simulink model "LQR_Controller"  (R2025a)
settings: Solver=VariableStepAuto  StartTime=0.0  StopTime=10.0  RelTol=1e-3
settings Model: Creator=xing2  LastModifiedBy=xing2

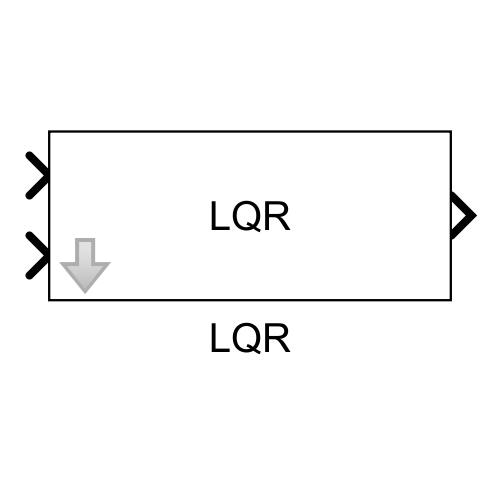
[thumbnail: Simulink's stored preview of the top-level diagram]
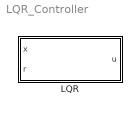
== system LQR_Controller ==
  LQR : Subsystem  mask{K_vec=[3 1], Ki=0, UL=10, LL=-10}
      mask prompts: K_vec "K vector"; Ki "Ki (integral)"; UL "Upper Limit"; LL "Lower Limit"
      mask help: LQR State Feedback Controller with integral action
      mask Display: disp('LQR');

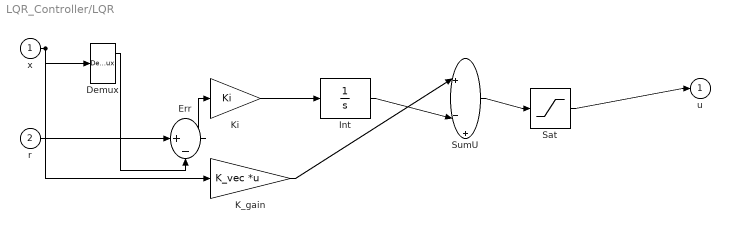
== system LQR_Controller/LQR ==
  x : Inport
  r : Inport  Port=2
  Demux : Demux  Outputs=2
  Err : Sum  Inputs=|+-
  Int : Integrator
  K_gain : Gain  Gain=K_vec  Multiplication=Matrix(K*u)
  Ki : Gain  Gain=Ki
  Sat : Saturate  UpperLimit=UL  LowerLimit=LL
  SumU : Sum  Inputs=|+-+
  u : Outport
  wires:
  x/1 -> Demux/1, K_gain/1
  r/1 -> Err/1
  Demux/1 -> Err/2
  Err/1 -> Ki/1
  Ki/1 -> Int/1
  K_gain/1 -> SumU/1
  Int/1 -> SumU/2
  SumU/1 -> Sat/1
  Sat/1 -> u/1
